simulink library "Lib_Piccolo"  (R2018b)
settings: Solver=VariableStepAuto  StartTime=0.0  StopTime=10.0  RelTol=1e-3
values from neighbouring files (symbols this model uses):
  AccelErrInt2Brakes = 0.15    [SimulationControlConfig16P.m]    (also in SimulationControlConfig16P_F0.m; SimulationControlConfig16P_F2.m; SimulationControlConfig16P_LEGACY.m; SimulationControlConfigTAILLESS.m = 0.2)
  AileronMax = 25    [SimulationControlConfig16P.m]    (also in SimulationControlConfig16P_F0.m; SimulationControlConfig16P_F2.m; SimulationControlConfig16P_LEGACY.m; SimulationControlConfigTAILLESS.m)
  AileronPower = 0.00268    [SimulationControlConfig16P.m]    (also in SimulationControlConfig16P_F0.m; SimulationControlConfig16P_F2.m; SimulationControlConfig16P_LEGACY.m; SimulationControlConfigTAILLESS.m = 0.002266)
  AileronSurfaceMax = 45    [SimulationControlConfig16P.m]    (also in SimulationControlConfig16P_F0.m; SimulationControlConfig16P_F2.m; SimulationControlConfig16P_LEGACY.m; SimulationControlConfigTAILLESS_CGAFT_F0.m = 25)
  AileronTrim = 0    [SimulationControlConfig16P.m]    (also in SimulationControlConfig16P_F0.m; SimulationControlConfig16P_F2.m; SimulationControlConfig16P_LEGACY.m; SimulationControlConfigTAILLESS.m)
  Alt = 1000 + TerrainHeight    [SimulationStateConfig.m]
  AltCruise_m = Alt * 0.3048    [SimulationControlConfig16P.m]    (also in SimulationControlConfig16P_F2.m; SimulationControlConfigTAILLESS.m = Alt/3.28084; SimulationControlConfigTAILLESS_CGAFT_F0.m = 640; SimulationControlConfigTAILLESS_CGFWD_F0.m = 640)
  AltitudeRate2PitchCmdIntegratorInit = 0.1    [SimulationControlPre.m]
  AltMax = 10000    [SimulationControlConfig16P.m]    (also in SimulationControlConfig16P_F0.m; SimulationControlConfig16P_F2.m; SimulationControlConfig16P_LEGACY.m; SimulationControlConfigTAILLESS.m)
  AltMaxAccel = 2.5    [SimulationControlConfig16P.m]    (also in SimulationControlConfig16P_F0.m = 2; SimulationControlConfig16P_F2.m = 2; SimulationControlConfig16P_LEGACY.m = 0.9; SimulationControlConfigTAILLESS.m = 2)
  AltMin = 0    [SimulationControlConfig16P.m]    (also in SimulationControlConfig16P_F0.m; SimulationControlConfig16P_F2.m; SimulationControlConfig16P_LEGACY.m; SimulationControlConfigTAILLESS.m)
  AltRateCmd2Pitch = 0.26    [SimulationControlConfig16P.m]    (also in SimulationControlConfig16P_F0.m = 0.35; SimulationControlConfig16P_F2.m = 0.35; SimulationControlConfig16P_LEGACY.m = 0.6; SimulationControlConfigTAILLESS.m = 0.9)
  AltRateError2Pitch = 0.34    [SimulationControlConfig16P.m]    (also in SimulationControlConfig16P_F0.m = 0.61; SimulationControlConfig16P_F2.m = 0.61; SimulationControlConfig16P_LEGACY.m = 0.4; SimulationControlConfigTAILLESS.m = 0.3)
  AltRateErrorInt2Pitch = 0.61    [SimulationControlConfig16P.m]    (also in SimulationControlConfig16P_F0.m = 0.28; SimulationControlConfig16P_F2.m = 0.28; SimulationControlConfig16P_LEGACY.m = 0.45; SimulationControlConfigTAILLESS.m = 0.15)
  AltRateLpfCutOff = 3    [SimulationControlConfig16P.m]    (also in SimulationControlConfig16P_F0.m; SimulationControlConfig16P_F2.m; SimulationControlConfig16P_LEGACY.m; SimulationControlConfigTAILLESS.m = 5)
  AutoNosegear2Rudder = 26    [SimulationControlConfig16P.m]    (also in SimulationControlConfig16P_F0.m; SimulationControlConfig16P_F2.m; SimulationControlConfig16P_LEGACY.m; SimulationControlConfigTAILLESS.m = 25.2)
  b = 5.54    [SimulationControlConfig16P.m]    (also in SimulationControlConfig16P_F0.m; SimulationControlConfig16P_F2.m; SimulationControlConfig16P_LEGACY.m; SimulationControlConfigTAILLESS.m = 2.37)
  Bank2AileronIntegratorInit = 0    [SimulationControlPre.m]
  BankMax_User = BankMax_User/180*pi    (= 0.610865238198)    [SimulationControlConfig16P.m]    (also in SimulationControlConfig16P_F0.m = 0.523598775598; SimulationControlConfig16P_F2.m = 0.523598775598; SimulationControlConfig16P_LEGACY.m = 0.523598775598; SimulationControlConfigTAILLESS.m = 0.558505360638)
  baseLegFlaps = 20    [SimulationControlConfig16P.m]    (also in SimulationControlConfig16P_F0.m; SimulationControlConfig16P_F2.m = 15; SimulationControlConfig16P_LEGACY.m = 0; SimulationControlConfigTAILLESS.m = 0)
  C = GeneticOpt.C    [SimulationCostFunction.m]
  c = Sw/b    (= 0.841696750903)    [SimulationControlConfig16P.m]    (also in SimulationControlConfig16P_F0.m; SimulationControlConfig16P_F2.m; SimulationControlConfig16P_LEGACY.m; SimulationControlConfigTAILLESS.m = 0.354008438819)
  cell2WheelFactorMG = 5.98    [SimulationSensorConfig16P_LEGACY.m]
  cell2WheelFactorNG = 1    [SimulationSensorConfig16P_LEGACY.m]
  cellSatMaxMG = 15000    [SimulationSensorConfig16P.m]    (also in SimulationSensorConfig16P_LEGACY.m; SimulationSensorConfigTAILLESS7P.m; SimulationSensorConfigUTAIL7P.m)
  cellSatMaxNG = 1000    [SimulationSensorConfig16P.m]    (also in SimulationSensorConfig16P_LEGACY.m; SimulationSensorConfigTAILLESS7P.m; SimulationSensorConfigUTAIL7P.m)
  cellSatMinMG = -15000    [SimulationSensorConfig16P.m]    (also in SimulationSensorConfig16P_LEGACY.m; SimulationSensorConfigTAILLESS7P.m; SimulationSensorConfigUTAIL7P.m)
  cellSatMinNG = -1000    [SimulationSensorConfig16P.m]    (also in SimulationSensorConfig16P_LEGACY.m; SimulationSensorConfigTAILLESS7P.m; SimulationSensorConfigUTAIL7P.m)
  CL_Limit = CL_Max    (= 0.54)    [SimulationControlConfig16P.m]    (also in SimulationControlConfig16P_F0.m; SimulationControlConfig16P_F2.m = 0.638; SimulationControlConfig16P_LEGACY.m; SimulationControlConfigTAILLESS.m = 0.525)
  CL_Max = 0.54    [SimulationControlConfig16P.m]    (also in SimulationControlConfig16P_F0.m; SimulationControlConfig16P_F2.m = 0.638; SimulationControlConfig16P_LEGACY.m; SimulationControlConfigTAILLESS.m = 0.525)
  CL_Max_Nom = 0.465    [SimulationControlConfig16P.m]    (also in SimulationControlConfig16P_F0.m; SimulationControlConfig16P_F2.m = 0.563; SimulationControlConfig16P_LEGACY.m; SimulationControlConfigTAILLESS.m = 0.39)
  CL_Min = 0    [SimulationControlConfig16P.m]    (also in SimulationControlConfig16P_F0.m; SimulationControlConfig16P_F2.m; SimulationControlConfig16P_LEGACY.m; SimulationControlConfigTAILLESS.m)
  ClimbMaxFraction = 0.35    [SimulationControlConfig16P.m]    (also in SimulationControlConfig16P_F0.m = 0.17; SimulationControlConfig16P_F2.m = 0.17; SimulationControlConfig16P_LEGACY.m = 0.24; SimulationControlConfigTAILLESS.m = 0.21)
  ClimboutMaxBank = 7.0    (= 7)    [SimulationControlConfig16P.m]    (also in SimulationControlConfig16P_F0.m; SimulationControlConfig16P_F2.m; SimulationControlConfig16P_LEGACY.m; SimulationControlConfigTAILLESS.m = 5)
  ClimboutTimer = 7.0    (= 7)    [SimulationControlConfig16P.m]    (also in SimulationControlConfig16P_F0.m; SimulationControlConfig16P_F2.m; SimulationControlConfig16P_LEGACY.m; SimulationControlConfigTAILLESS.m)
  dCl_per_dFlap = 0.005581818    [SimulationControlConfig16P.m]    (also in SimulationControlConfig16P_F0.m = 0; SimulationControlConfig16P_F2.m = 0.0065; SimulationControlConfig16P_LEGACY.m = 0; SimulationControlConfigTAILLESS.m = 0)
  DecelerationCmd = 3.1    [SimulationControlConfig16P.m]    (also in SimulationControlConfig16P_F0.m; SimulationControlConfig16P_F2.m; SimulationControlConfig16P_LEGACY.m; SimulationControlConfigTAILLESS.m = 0.1)
  DeRotateLogicEndTimer = abs((NoseDownLimit_Deg-1)/DeRotateRamp_Dps)    [SimulationControlConfig16P.m]    (also in SimulationControlConfig16P_F0.m; SimulationControlConfig16P_F2.m; SimulationControlConfig16P_LEGACY.m; SimulationControlConfigTAILLESS.m)
  DeRotateLogicHoldNoseUpTimer = 0.1    [SimulationControlConfig16P.m]    (also in SimulationControlConfig16P_F0.m; SimulationControlConfig16P_F2.m; SimulationControlConfig16P_LEGACY.m; SimulationControlConfigTAILLESS.m)
  DeRotateLogicTimerTimeout = 2    [SimulationControlConfig16P.m]    (also in SimulationControlConfig16P_F0.m; SimulationControlConfig16P_F2.m; SimulationControlConfig16P_LEGACY.m; SimulationControlConfigTAILLESS.m)
  DeRotateLowerCmdSaturation = 0    [SimulationControlConfig16P.m]    (also in SimulationControlConfig16P_F0.m; SimulationControlConfig16P_F2.m; SimulationControlConfig16P_LEGACY.m; SimulationControlConfigTAILLESS.m)
  DeRotateRamp_Dps = 3    [SimulationControlConfig16P.m]    (also in SimulationControlConfig16P_F0.m; SimulationControlConfig16P_F2.m; SimulationControlConfig16P_LEGACY.m; SimulationControlConfigTAILLESS.m = 8)
  DeRotateUpperCmdSaturation = 7    [SimulationControlConfig16P.m]    (also in SimulationControlConfig16P_F0.m; SimulationControlConfig16P_F2.m; SimulationControlConfig16P_LEGACY.m; SimulationControlConfigTAILLESS.m)
  DescentMaxFraction = 0.22    [SimulationControlConfig16P.m]    (also in SimulationControlConfig16P_F0.m = 0.2; SimulationControlConfig16P_F2.m = 0.2; SimulationControlConfig16P_LEGACY.m = 0.2; SimulationControlConfigTAILLESS.m = 0.17)
  DesktopSimTerrainOffset_m = 0.406    [SimulationAircraftConfig.m]
  downwindFlaps = 0    [SimulationControlConfig16P.m]    (also in SimulationControlConfig16P_F0.m; SimulationControlConfig16P_F2.m = 15; SimulationControlConfig16P_LEGACY.m; SimulationControlConfigTAILLESS.m)
  downwindSplitAil = 0    [SimulationControlConfig16P_F2.m]
  DP_init = 0.5*1.225*V_init^2    [SimulationControlConfig16P.m]    (also in SimulationControlConfig16P_F0.m; SimulationControlConfig16P_F2.m; SimulationControlConfig16P_LEGACY.m; SimulationControlConfigTAILLESS.m)
  dscNoiseMG = 1    [SimulationSensorConfig16P_LEGACY.m]
  dscNoiseNG = 0.25    [SimulationSensorConfig16P_LEGACY.m]
  DSCnumBits = 24    [SimulationSensorConfig16P.m]    (also in SimulationSensorConfig16P_LEGACY.m; SimulationSensorConfigTAILLESS7P.m; SimulationSensorConfigUTAIL7P.m)
  DSCRangeMaxMG = 15000    [SimulationSensorConfig16P.m]    (also in SimulationSensorConfig16P_LEGACY.m; SimulationSensorConfigTAILLESS7P.m; SimulationSensorConfigUTAIL7P.m)
  DSCRangeMaxNG = 1000    [SimulationSensorConfig16P.m]    (also in SimulationSensorConfig16P_LEGACY.m; SimulationSensorConfigTAILLESS7P.m; SimulationSensorConfigUTAIL7P.m)
  DSCRangeMinMG = -15000    [SimulationSensorConfig16P.m]    (also in SimulationSensorConfig16P_LEGACY.m; SimulationSensorConfigTAILLESS7P.m; SimulationSensorConfigUTAIL7P.m)
  DSCRangeMinNG = -1000    [SimulationSensorConfig16P.m]    (also in SimulationSensorConfig16P_LEGACY.m; SimulationSensorConfigTAILLESS7P.m; SimulationSensorConfigUTAIL7P.m)
  dt = DLLSim.dt    [SimulationTimeStep.m]    (also in SimulationTrim.m = 0.02)
  EarlyTouchdownThreshold = 3.0    (= 3)    [SimulationControlConfig16P.m]    (also in SimulationControlConfig16P_F0.m; SimulationControlConfig16P_F2.m; SimulationControlConfig16P_LEGACY.m; SimulationControlConfigTAILLESS.m)
  ElevatorDeflectionRate = 15    [SimulationControlConfig16P.m]    (also in SimulationControlConfig16P_F0.m; SimulationControlConfig16P_F2.m; SimulationControlConfig16P_LEGACY.m = 12; SimulationControlConfigTAILLESS.m = 5)
  ElevatorMax = 25    [SimulationControlConfig16P.m]    (also in SimulationControlConfig16P_F0.m; SimulationControlConfig16P_F2.m; SimulationControlConfig16P_LEGACY.m; SimulationControlConfigTAILLESS.m)
  ElevatorPower = -0.002209    [SimulationControlConfig16P.m]    (also in SimulationControlConfig16P_F0.m; SimulationControlConfig16P_F2.m; SimulationControlConfig16P_LEGACY.m; SimulationControlConfigTAILLESS.m = -0.002668)
  ElevatorTrim = -3.5    [SimulationControlConfig16P.m]    (also in SimulationControlConfig16P_F0.m; SimulationControlConfig16P_F2.m; SimulationControlConfig16P_LEGACY.m; SimulationControlConfigTAILLESS.m = -3)
  elevonBias = 0    [SimulationControlConfig16P.m]    (also in SimulationControlConfig16P_F0.m; SimulationControlConfig16P_F2.m; SimulationControlConfig16P_LEGACY.m; SimulationControlConfigTAILLESS.m)
  Enable_TAS_Protection = 0    [SimulationControlConfig16P.m]    (also in SimulationControlConfig16P_F0.m; SimulationControlConfig16P_F2.m; SimulationControlConfig16P_LEGACY.m; SimulationControlConfigTAILLESS.m)
  EnableCrossTrackAbort = 1    [SimulationControlConfig16P.m]    (also in SimulationControlConfigTAILLESS.m; SimulationControlConfigTAILLESS_CGAFT_F0.m; SimulationControlConfigTAILLESS_CGFWD_F0.m; SimulationControlConfigTAILLESS_CGFWD_F2.m)
  EnergyBandwidth = 0.04    [SimulationControlConfig16P.m]    (also in SimulationControlConfig16P_F0.m = 0.03; SimulationControlConfig16P_F2.m = 0.03; SimulationControlConfig16P_LEGACY.m = 0.02; SimulationControlConfigTAILLESS.m = 0.06)
  EngineLhFuelCut = 0    [SimulationAircraftConfig.m]
  EngineRhFuelCut = 0    [SimulationAircraftConfig.m]
  FastThrottleRate = 0.075    [SimulationControlConfig16P.m]    (also in SimulationControlConfig16P_F0.m = 0.05; SimulationControlConfig16P_F2.m = 0.05; SimulationControlConfig16P_LEGACY.m = 0.05; SimulationControlConfigTAILLESS.m = 0.1)
  FilterWarmUpTime = 2    [SimulationSensorConfig16P.m]    (also in SimulationSensorConfig16P_LEGACY.m; SimulationSensorConfigTAILLESS7P.m; SimulationSensorConfigUTAIL7P.m)
  finalApproachFlaps = 20    [SimulationControlConfig16P.m]    (also in SimulationControlConfig16P_F0.m; SimulationControlConfig16P_F2.m = 15; SimulationControlConfig16P_LEGACY.m = 0; SimulationControlConfigTAILLESS.m = 0)
  finalApproachSplitAil = 20    [SimulationControlConfig16P_F2.m]
  FinalDescentSlope_Deg = testPlans(testIndx).descentSlope    [SimulationControlConfig16P.m]    (also in SimulationControlConfig16P_F0.m; SimulationControlConfig16P_F2.m; SimulationControlConfig16P_LEGACY.m; SimulationControlConfigTAILLESS.m)
  flapMax = 0    [SimulationControlConfig16P.m]    (also in SimulationControlConfig16P_F0.m = 35; SimulationControlConfig16P_F2.m = 33; SimulationControlConfig16P_LEGACY.m; SimulationControlConfigTAILLESS.m)
  flapRate = 7.5    [SimulationControlConfig16P.m]    (also in SimulationControlConfig16P_F0.m; SimulationControlConfig16P_F2.m; SimulationControlConfig16P_LEGACY.m; SimulationControlConfigTAILLESS.m = 6.6)
  FlareHeight = 5    [SimulationControlConfig16P.m]    (also in SimulationControlConfig16P_F0.m; SimulationControlConfig16P_F2.m; SimulationControlConfig16P_LEGACY.m = 4.8; SimulationControlConfigTAILLESS.m = 2.75)
  FlareVerticalRate_mps = -0.4    [SimulationControlConfig16P.m]    (also in SimulationControlConfig16P_F0.m; SimulationControlConfig16P_F2.m; SimulationControlConfig16P_LEGACY.m = -0.5; SimulationControlConfigTAILLESS.m = -0.15)
  Fp_Aileron = 0.55*2*pi*RollRateLpfCutoff*dt    [SimulationControlConfig16P.m]    (also in SimulationControlConfig16P_F0.m; SimulationControlConfig16P_F2.m; SimulationControlConfig16P_LEGACY.m; SimulationControlConfigTAILLESS.m)
  Fp_Alt = 2*pi*0.55*AltBandwidth    (= 0.622035345411)    [SimulationControlConfig16P.m]    (also in SimulationControlConfig16P_F0.m; SimulationControlConfig16P_F2.m; SimulationControlConfig16P_LEGACY.m = 0.099; SimulationControlConfigTAILLESS.m = 0.207345115137)
  Fp_AltRate = 0.55*2*pi*AltRateLpfCutOff*dt    [SimulationControlConfig16P.m]    (also in SimulationControlConfig16P_F0.m; SimulationControlConfig16P_F2.m; SimulationControlConfig16P_LEGACY.m; SimulationControlConfigTAILLESS.m)
  Fp_Elevator = 0.55*2*pi*PitchRateLpfCutoff*dt    [SimulationControlConfig16P.m]    (also in SimulationControlConfig16P_F0.m; SimulationControlConfig16P_F2.m; SimulationControlConfig16P_LEGACY.m; SimulationControlConfigTAILLESS.m)
  Fp_Energy = 0.55*2*pi*EnergyBandwidth    (= 0.138230076758)    [SimulationControlConfig16P.m]    (also in SimulationControlConfig16P_F0.m = 0.103672557568; SimulationControlConfig16P_F2.m = 0.103672557568; SimulationControlConfig16P_LEGACY.m = 0.069115038379; SimulationControlConfigTAILLESS.m = 0.207345115137)
  Fp_Energy2 = 0.55*2*pi*EnergyBandwidth*dt    [SimulationControlConfig16P.m]    (also in SimulationControlConfig16P_F0.m; SimulationControlConfig16P_F2.m; SimulationControlConfig16P_LEGACY.m; SimulationControlConfigTAILLESS.m)
  Fp_Pitch = 0.55*2*pi*PitchBandwidth    (= 2.45358386245)    [SimulationControlConfig16P.m]    (also in SimulationControlConfig16P_F0.m; SimulationControlConfig16P_F2.m = 1.72787595947; SimulationControlConfig16P_LEGACY.m = 3.11017672705; SimulationControlConfigTAILLESS.m = 1.55508836353)
  Fp_Pitch_2 = 0.55*2*pi*PitchBandwidth*dt    [SimulationControlConfig16P.m]    (also in SimulationControlConfig16P_F0.m; SimulationControlConfig16P_F2.m; SimulationControlConfig16P_LEGACY.m; SimulationControlConfigTAILLESS.m)
  Fp_Roll = RollBandwidth^2    (= 1.69)    [SimulationControlConfig16P.m]    (also in SimulationControlConfig16P_F0.m = 1.44; SimulationControlConfig16P_F2.m = 1.44; SimulationControlConfig16P_LEGACY.m = 1.44; SimulationControlConfigTAILLESS.m = 1.21)
  Fp_Rudder = 0.55*2*pi*YawRateLpfCutoff*dt    [SimulationControlConfig16P.m]    (also in SimulationControlConfig16P_F0.m; SimulationControlConfig16P_F2.m; SimulationControlConfig16P_LEGACY.m; SimulationControlConfigTAILLESS.m)
  Fp_TAS = 0.55*2*pi*TASBandwidth    (= 0.103672557568)    [SimulationControlConfig16P.m]    (also in SimulationControlConfig16P_F0.m; SimulationControlConfig16P_F2.m; SimulationControlConfig16P_LEGACY.m; SimulationControlConfigTAILLESS.m = 0.172787595947)
  Fp_TAS_Filter = 2*pi*TasLpfCutoff*dt    [SimulationControlConfig16P.m]    (also in SimulationControlConfig16P_F0.m; SimulationControlConfig16P_F2.m; SimulationControlConfig16P_LEGACY.m; SimulationControlConfigTAILLESS.m)
  Fp_Turn = 0.55*2*pi*TurnErrLPFcutoff    (= 0.172787595947)    [SimulationControlConfig16P.m]    (also in SimulationControlConfig16P_F0.m = 0.0345575191895; SimulationControlConfig16P_F2.m = 0.0345575191895; SimulationControlConfig16P_LEGACY.m = 0.0345575191895; SimulationControlConfigTAILLESS.m)
  Fp_TurnDerr = 0.55*2*pi*TurnDerivativeLPFcutoff    (= 0.172787595947)    [SimulationControlConfig16P.m]    (also in SimulationControlConfig16P_F0.m = 0.0345575191895; SimulationControlConfig16P_F2.m = 0.0345575191895; SimulationControlConfig16P_LEGACY.m = 0.0345575191895; SimulationControlConfigTAILLESS.m)
  FTV = 3    [SimulationAircraftConfig.m]
  ftvStaticPositionError = 1/1.18    (= 0.847457627119)    [SimulationSensorConfig16P.m]    (also in SimulationSensorConfig16P_LEGACY.m; SimulationSensorConfigTAILLESS7P.m = 1; SimulationSensorConfigUTAIL7P.m = 1)
  g = 9.81    [SimulationStateConfig.m]
  goAroundSplitAil = 0    [SimulationControlConfig16P_F2.m]
  GustSpd_Kts = testPlans(testIndx).gustSpd    [SimulationStateConfig.m]
  GustTriggerVal = testPlans(testIndx).gustTriggerVal    [SimulationStateConfig.m]
  HeadingErr2TurnRate = 0.5    [SimulationControlConfig16P.m]    (also in SimulationControlConfig16P_F0.m; SimulationControlConfig16P_F2.m; SimulationControlConfig16P_LEGACY.m; SimulationControlConfigTAILLESS.m)
  HeadingErrDer2TurnRate = 0.3    [SimulationControlConfig16P.m]    (also in SimulationControlConfig16P_F0.m; SimulationControlConfig16P_F2.m; SimulationControlConfig16P_LEGACY.m; SimulationControlConfigTAILLESS.m)
  IASbounce = IASstall*0.8    [SimulationControlPre.m]
  IAScruiseCMD = sqrt(2*m*9.81/(1.225*Sw*CL_cruise))    [SimulationControlConfig16P.m]    (also in SimulationControlConfig16P_F0.m; SimulationControlConfig16P_F2.m; SimulationControlConfig16P_LEGACY.m; SimulationControlConfigTAILLESS.m)
  IASfinalCMD = 1.12 * IASmin    [SimulationControlConfig16P.m]    (also in SimulationControlConfig16P_F0.m = 1.14 * IASmin; SimulationControlConfig16P_F2.m = 1.10 * IASmin; SimulationControlConfig16P_LEGACY.m = 1.10 * IASmin; SimulationControlConfigTAILLESS.m = 1.14 * IASmin)
  IASflareCMD = IASstall    [SimulationControlConfig16P.m]    (also in SimulationControlConfig16P_F0.m; SimulationControlConfig16P_F2.m; SimulationControlConfig16P_LEGACY.m; SimulationControlConfigTAILLESS.m)
  IASmax = 64    [SimulationControlConfig16P.m]    (also in SimulationControlConfig16P_F0.m = 46; SimulationControlConfig16P_F2.m = 52; SimulationControlConfig16P_LEGACY.m = 46; SimulationControlConfigTAILLESS.m = 38.9)
  IASmin = sqrt(2*m*9.81/(1.225*Sw*0.9*CL_Max_Nom))    [SimulationControlConfig16P.m]    (also in SimulationControlConfig16P_F0.m; SimulationControlConfig16P_F2.m; SimulationControlConfig16P_LEGACY.m; SimulationControlConfigTAILLESS.m)
  IASshortCMD = IASstall    [SimulationControlConfig16P.m]    (also in SimulationControlConfig16P_F0.m; SimulationControlConfig16P_F2.m; SimulationControlConfig16P_LEGACY.m; SimulationControlConfigTAILLESS.m)
  IASstall = sqrt(2*m*9.81/(1.225*Sw*CL_Max))    [SimulationControlConfig16P.m]    (also in SimulationControlConfig16P_F0.m; SimulationControlConfig16P_F2.m; SimulationControlConfig16P_LEGACY.m; SimulationControlConfigTAILLESS.m)
  inFlight = 1    [SimulationControlConfig16P.m]    (also in SimulationControlConfigTAILLESS.m; SimulationControlConfigTAILLESS_CGAFT_F0.m; SimulationControlConfigTAILLESS_CGFWD_F0.m; SimulationControlConfigTAILLESS_CGFWD_F2.m)
  JetCatOffset = 5    [SimulationControlConfig16P.m]    (also in SimulationControlConfig16P_F0.m; SimulationControlConfig16P_F2.m; SimulationControlConfig16P_LEGACY.m)
  LaunchRollingElevator = -1.5    [SimulationControlConfig16P.m]    (also in SimulationControlConfig16P_F0.m; SimulationControlConfig16P_F2.m = 1.25; SimulationControlConfig16P_LEGACY.m; SimulationControlConfigTAILLESS.m = 1)
  ldg_NosegearMax = 10    [SimulationControlConfig16P.m]    (also in SimulationControlConfig16P_F0.m; SimulationControlConfig16P_F2.m; SimulationControlConfig16P_LEGACY.m; SimulationControlConfigTAILLESS.m)
  ldg_TrackVyErrInt2Nosegear = 0.1250    (= 0.125)    [SimulationControlConfig16P.m]    (also in SimulationControlConfig16P_F0.m; SimulationControlConfig16P_F2.m; SimulationControlConfig16P_LEGACY.m; SimulationControlConfigTAILLESS.m = 0.00714285714286)
  ldg_TrackVyErrPro2Nosegear = 0.35    [SimulationControlConfig16P.m]    (also in SimulationControlConfig16P_F0.m; SimulationControlConfig16P_F2.m; SimulationControlConfig16P_LEGACY.m; SimulationControlConfigTAILLESS.m = 0.0546666666667)
  ldg_TrackY2Vy = 0.07    [SimulationControlConfig16P.m]    (also in SimulationControlConfig16P_F0.m; SimulationControlConfig16P_F2.m; SimulationControlConfig16P_LEGACY.m; SimulationControlConfigTAILLESS.m = 0.17)
  ldg_Vy2NosegearScalingPower = 1.075    [SimulationControlConfig16P.m]    (also in SimulationControlConfig16P_F0.m; SimulationControlConfig16P_F2.m; SimulationControlConfig16P_LEGACY.m; SimulationControlConfigTAILLESS.m = 0.6)
  ldg_Y2VyScalingPower = 0.175    [SimulationControlConfig16P.m]    (also in SimulationControlConfig16P_F0.m; SimulationControlConfig16P_F2.m; SimulationControlConfig16P_LEGACY.m; SimulationControlConfigTAILLESS.m = 0)
  ldg_YawRate2Nosegear = 0.175    [SimulationControlConfig16P.m]    (also in SimulationControlConfig16P_F0.m; SimulationControlConfig16P_F2.m; SimulationControlConfig16P_LEGACY.m; SimulationControlConfigTAILLESS.m = 0.065)
  LiftSlope = 0.064285    [SimulationControlConfig16P.m]    (also in SimulationControlConfig16P_F0.m; SimulationControlConfig16P_F2.m; SimulationControlConfig16P_LEGACY.m; SimulationControlConfigTAILLESS.m = 0.058631)
  LPFaileronInit = 0    [SimulationControlPre.m]
  LPFclestInit = 0    [SimulationControlPre.m]
  LPFenergyFFInit = 0    [SimulationControlPre.m]
  ... (+122 more)
undefined symbols (not defined in the file or in its folder): abortFlag, alphaHPF, apmDelay, BRWNOUT, CRAWOR, CRAWUR, DiscIntNeverNeededParam, DLLSim, DLLSimStep, ECOMOR, ECOMUR, Fp_Tas, GustTrigger_HeightAgl_m, IPSTAT, LCINTEG, Ldg_Persist_Time, LOWER_FLAGS, MSG_ENABLE, NoiseStd, OLDVAL, OVERRIDE_ENABLE, OVERRIDE_VALUE, REBOOT, reversionEnable, revIASMax, revIASMin, revPitchMax, revPitchMin, revPitchRateMax, revRollMax, revRollRateMax, SAMPLE, SCALON, SensorModel, sigbuilder_block, Sim_Vx, Sim_Vy, Sim_Vz, Sim_Xpos, Sim_Ypos, Sim_Zpos, SYSOR, SYSUR, TARE, TEMPOR, TEMPUR, testIndx, testPlan, testPlans, Trim_piccoloInCmd, Trim_REFSI_FD_IN_nmodeCgShifterCmd_Flag, Trim_REFSI_FD_IN_nmodeCgShifterCmd_Ft, Trim_REFSI_FD_IN_nmodeCgShifterCmdType, Trim_REFSI_FD_IN_nmodeCgShifterNRCActive, Trim_REFSI_FD_IN_nmodeFlapLhIBCmd_Deg, Trim_REFSI_FD_IN_nmodeFlapLhOBCmd_Deg, Trim_REFSI_FD_IN_nmodeFlapRhIBCmd_Deg, Trim_REFSI_FD_IN_nmodeFlapRhOBCmd_Deg, Trim_REFSI_FD_IN_nmodeSlatLhCmd_Deg ... (+11)
libraries: simulink x1237, $bdroot x179, aerolibconvert2 x63, dspswit3 x25, aerolibatmos2 x5, simulink_extras x4, dsparch4 x2, Lib_Piccolo_Alt x2, eeGeneralControl x1, dspindex x1
(part 5 of 74)

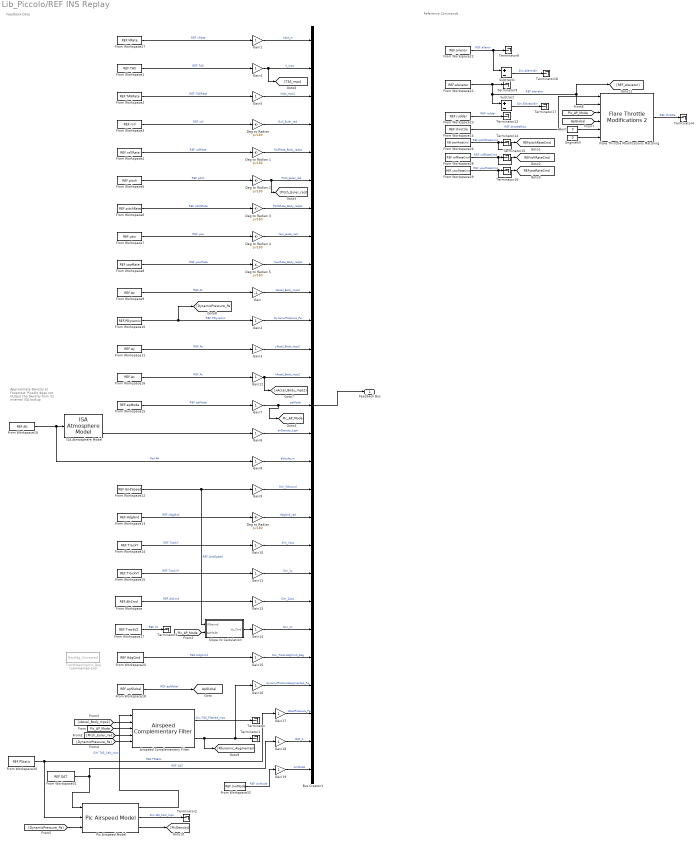
== system Lib_Piccolo/REF INS Replay ==
  note: Feedback Data
  note: Approximate Density at Foremost. Piccolo does not Output the Density from its internal ISA lookup
  note: Reference Commands
  Abort : Constant  Value=0
  Airspeed Complementary Filter : $bdroot/Airspeed Complementary Filter  SystemSampleTime=-1
  Bus Creator1 : BusCreator  Inputs=27
  Deg to Radian : Gain  Gain=pi/180
  Deg to Radian {,1..5} (6 alike) : Gain  Gain=pi/180
  EngineKill : Constant  Value=0
  Flare Throttle Modifications Matching : $bdroot/Throttle Control (Alt Mode)/Flare Throttle Modifications 2  SystemSampleTime=-1
  From Workspace : FromWorkspace  VariableName=REF.AltCmd  SampleTime=0
  From Workspace1 : FromWorkspace  VariableName=REF.TAS  SampleTime=0
  From Workspace10 : FromWorkspace  VariableName=REF.PDynamic  SampleTime=0
  From Workspace11 : FromWorkspace  VariableName=REF.Ay  SampleTime=0
  From Workspace12 : FromWorkspace  VariableName=REF.GndSpeed  SampleTime=0
  From Workspace13 : FromWorkspace  VariableName=REF.HdgGnd  SampleTime=0
  From Workspace14 : FromWorkspace  VariableName=REF.TrackY  SampleTime=0
  From Workspace15 : FromWorkspace  VariableName=REF.TrackVY  SampleTime=0
  From Workspace16 : FromWorkspace  VariableName=REF.Ax  SampleTime=0
  From Workspace17 : FromWorkspace  VariableName=REF.TrackVZ  SampleTime=0
  From Workspace18 : FromWorkspace  VariableName=REF.apGlobal  SampleTime=0
  From Workspace19 : FromWorkspace  VariableName=REF.Alt  SampleTime=0
  From Workspace2 : FromWorkspace  VariableName=REF.TASRate  SampleTime=0
  From Workspace20 : FromWorkspace  VariableName=REF.HdgCmd  SampleTime=0
  From Workspace21 : FromWorkspace  VariableName=REF.elevator  SampleTime=0
  From Workspace22 : FromWorkspace  VariableName=REF.aileron  SampleTime=0
  From Workspace23 : FromWorkspace  VariableName=REF.rudder  SampleTime=0
  From Workspace24 : FromWorkspace  VariableName=REF.throttle  SampleTime=0
  From Workspace25 : FromWorkspace  VariableName=REF.apMode  SampleTime=0
  From Workspace26 : FromWorkspace  VariableName=REF.pitchRateCmd  SampleTime=0
  From Workspace27 : FromWorkspace  VariableName=REF.VRate  SampleTime=0
  From Workspace28 : FromWorkspace  VariableName=REF.rollRateCmd  SampleTime=0
  From Workspace29 : FromWorkspace  VariableName=REF.yawRateCmd  SampleTime=0
  From Workspace3 : FromWorkspace  VariableName=REF.roll  SampleTime=0
  From Workspace30 : FromWorkspace  VariableName=REF.PStatic  SampleTime=0
  From Workspace31 : FromWorkspace  VariableName=REF.OAT  SampleTime=0
  From Workspace32 : FromWorkspace  VariableName=REF.lonMode  SampleTime=0
  From Workspace4 : FromWorkspace  VariableName=REF.rollRate  SampleTime=0
  From Workspace5 : FromWorkspace  VariableName=REF.pitch  SampleTime=0
  From Workspace6 : FromWorkspace  VariableName=REF.pitchRate  SampleTime=0
  From Workspace7 : FromWorkspace  VariableName=REF.yaw  SampleTime=0
  From Workspace8 : FromWorkspace  VariableName=REF.yawRate  SampleTime=0
  From Workspace9 : FromWorkspace  VariableName=REF.Az  SampleTime=0
  Gain : Gain  Gain=-1
  Gain{1..19} (19 alike) : Gain
  ISA Atmosphere Model : aerolibatmos2/ISA Atmosphere Model  custom=off  g=9.80665  gamma=1.4  R=287.0531  L=0.0065  h_trop=11000  h_strat=20000  rho0=1.225  P0=101325  T0=288.15  h0=0
      settings: SourceProductName=Aerospace Blockset
  Pic Airspeed Model : $bdroot/Pic Airspeed Model  correction=1
  Slope Vz Calculation : Subsystem
  Subtract : Sum  Inputs=+-
  Subtract1 : Sum  Inputs=+-
  Terminator{,1..4,8..9,12,14..18} (13 alike) : Terminator
  TrackHeadingInit_Deg : Constant  Commented=on  Value=RwyHdg_Corrected
  Feedback Bus : Outport
  tag scope: ApGlobal=global, Pic_AP_Mode=global, REFpitchRateCmd=global, REFrollRateCmd=global, REFyawRateCmd=global
  wires:
  Deg to Radian 2/1 -> [Pitch_Euler_rad], Bus Creator1/6  "Pitch_Euler_rad"
  Deg to Radian 3/1 -> Bus Creator1/7  "PitchRate_Body_radps"
  Gain/1 -> Bus Creator1/10  "zAccel_Body_mps2"
  Deg to Radian 5/1 -> Bus Creator1/9  "YawRate_Body_radps"
  Deg to Radian 4/1 -> Bus Creator1/8  "Yaw_Euler_rad"
  Bus Creator1/1 -> Feedback Bus/1
  Gain3/1 -> Bus Creator1/12  "yAccel_Body_mps2"
  Gain1/1 -> Bus Creator1/1  "hdot_m"
  Gain4/1 -> [TAS_mps], Bus Creator1/2  "V_mps"
  Gain5/1 -> Bus Creator1/3  "Vdot_mps2"
  "Deg to Radian "/1 -> Bus Creator1/4  "Roll_Euler_rad"
  Deg to Radian 1/1 -> Bus Creator1/5  "RollRate_Body_radps"
  Gain6/1 -> Bus Creator1/15  "airDensity_kgm"
  From Workspace27/1 -> Gain1/1  "REF.vRate"
  From Workspace2/1 -> Gain5/1  "REF.TASRate"
  From Workspace3/1 -> "Deg to Radian "/1  "REF.roll"
  From Workspace4/1 -> Deg to Radian 1/1  "REF.rollRate"
  From Workspace5/1 -> Deg to Radian 2/1  "REF.pitch"
  From Workspace6/1 -> Deg to Radian 3/1  "REF.pitchRate"
  From Workspace7/1 -> Deg to Radian 4/1  "REF.yaw"
  From Workspace8/1 -> Deg to Radian 5/1  "REF.yawRate"
  From Workspace9/1 -> Gain/1  "REF.Az"
  From Workspace10/1 -> [DynamicPressure_Pa], Gain2/1  "REF.PDynamic"
  From Workspace11/1 -> Gain3/1  "REF.Ay"
  ISA Atmosphere Model/4 -> Gain6/1
  From Workspace19/1 -> Gain8/1, ISA Atmosphere Model/1  "Ref.Alt"
  Gain7/1 -> [Pic_AP_Mode], Bus Creator1/14  "apMode"
  From Workspace25/1 -> Gain7/1  "REF.apMode"
  Gain8/1 -> Bus Creator1/16  "altitude_m"
  Gain9/1 -> Bus Creator1/17  "Sim_VGround"
  From Workspace12/1 -> Slope Vz Calculation/1(VGround), Gain9/1  "REF.GndSpeed"
  From Workspace13/1 -> Deg to Radian/1  "REF.HdgGnd"
  Deg to Radian/1 -> Bus Creator1/18  "HdgGnd_rad"
  From Workspace1/1 -> Gain4/1  "REF.TAS"
  From Workspace14/1 -> Gain10/1  "REF.TrackY"
  Gain10/1 -> Bus Creator1/19  "Sim_Ypos"
  From Workspace15/1 -> Gain11/1  "REF.TrackVY"
  Gain11/1 -> Bus Creator1/20  "Sim_Vy"
  From Workspace16/1 -> Gain12/1  "REF.Ax"
  Gain12/1 -> [xAccel_Body_mps2], Bus Creator1/13  "xAccel_Body_mps2"
  From Workspace/1 -> Gain13/1  "REF.AltCmd"
  Gain13/1 -> Bus Creator1/21  "Sim_Zpos"
  Gain14/1 -> Bus Creator1/22  "Sim_Vz"
  From Workspace17/1 -> Terminator3/1  "REF.Vz"
  From Workspace18/1 -> [ApGlobal]  "REF.apGlobal"
  Gain15/1 -> Bus Creator1/23  "Sim_TrackHdgCmd_Deg"
  From Workspace20/1 -> Gain15/1  "REF.HdgCmd"
  [Pic_AP_Mode] -> Airspeed Complementary Filter/3
  [Pitch_Euler_rad] -> Airspeed Complementary Filter/4
  [xAccel_Body_mps2] -> Airspeed Complementary Filter/2
  Airspeed Complementary Filter/1 -> Terminator/1  "Sim.TAS_Filtered_mps"
  [DynamicPressure_Pa] -> Airspeed Complementary Filter/5
  Airspeed Complementary Filter/2 -> [Pdynamic_Augmented], Gain16/1, Terminator1/1
  Gain16/1 -> Bus Creator1/24  "dynamicPressureAugmented_Pa"
  Pic Airspeed Model/1 -> Airspeed Complementary Filter/1  "Sim.TAS_Calc_mps"
  Pic Airspeed Model/2 -> Terminator2/1  "Sim.IAS_Calc_mps"
  [DynamicPressure_Pa] -> Pic Airspeed Model/3
  From Workspace30/1 -> Pic Airspeed Model/2, Gain17/1  "REF.PStatic"
  Gain17/1 -> Bus Creator1/25  "staticPressure_Pa"
  From Workspace31/1 -> Pic Airspeed Model/1, Gain18/1  "REF.OAT"
  Gain18/1 -> Bus Creator1/26  "OAT_C"
  Gain2/1 -> Bus Creator1/11  "DynamicPressure_Pa"
  Pic Airspeed Model/3 -> [PicDensity]
  Slope Vz Calculation/1(Vz_Cmd) -> Gain14/1
  [Pic_AP_Mode] -> Slope Vz Calculation/2(apMode)
  From Workspace24/1 -> Flare Throttle Modifications Matching/1  "REF.throttleRaw"
  Abort/1 -> Flare Throttle Modifications Matching/5
  From Workspace26/1 -> [REFpitchRateCmd], Terminator14/1  "REF.pitchRateCmd"
  From Workspace23/1 -> Terminator12/1  "REF.rudder"
  From Workspace29/1 -> [REFyawRateCmd], Terminator16/1  "REF.yawRateCmd"
  Subtract/1 -> Terminator17/1  "Sim.ElevatorErr"
  [Pic_AP_Mode] -> Flare Throttle Modifications Matching/3
  EngineKill/1 -> Flare Throttle Modifications Matching/6
  From Workspace22/1 -> Terminator8/1, Subtract1/1  "REF.aileron"
  Subtract1/1 -> Terminator18/1  "Sim.AileronErr"
  From Workspace21/1 -> Terminator9/1, [REF_elevator], Flare Throttle Modifications Matching/2, Subtract/1  "REF.elevator"
  Flare Throttle Modifications Matching/1 -> Terminator4/1  "REF.throttle"
  From Workspace28/1 -> [REFrollRateCmd], Terminator15/1  "REF.rollRateCmd"
  [ApGlobal] -> Flare Throttle Modifications Matching/4
  From Workspace32/1 -> Gain19/1  "REF.lonMode"
  Gain19/1 -> Bus Creator1/27  "lonMode"

== system Lib_Piccolo/Sliding Window Maximum ==
  note: Insert new element
  note: Remove last element
  note: Define dimensions
      | (initial conditions)
  windowInput : Inport
  IC : InitialCondition  Value=[zeros(N,1)]
  Max : MinMax  Function=max
  Memory : Memory
  Mux : Mux  Inputs=2
  Variable Selector : dspindex/Variable Selector  NumInputs=1  rowsOrCols=Rows  IdxMode=Fixed  Elements=1:N-1  ZerOneIdxMode=One-based  errmode=Clip Index  FillMode=on  FillValues=0
  windowMax : Outport
  wires:
  Memory/1 -> IC/1
  Mux/1 -> Max/1, Memory/1
  windowInput/1 -> Mux/1
  Variable Selector/1 -> Mux/2
  IC/1 -> Variable Selector/1
  Max/1 -> windowMax/1

== system Lib_Piccolo/Steering Controller Landing ==
  Y command : Inport
  Feedback : Inport  Port=2
  Bus Selector : BusSelector  OutputSignals=Sim_VGround,Sim_Ypos,Sim_Vy,YawRate_Body_radps
  Constant : Constant  Value=0
  Constant1 : Constant  Value=0
  Gain3 : Gain  Gain=1/4
  Gain4 : Gain  Gain=-1
  Integrator1 : Integrator  ExternalReset=level
  NOT : Logic  Operator=NOT  IconShape=distinctive  AllPortsSameDT=off  OutDataTypeStr=boolean
  "Nosegear rudder mixer " : Subsystem
  Nosegear scaling based on ground speed : Subsystem
  Product2 : Product
  Product3 : Product
  Saturation Dynamic1 : simulink/Discontinuities/Saturation Dynamic  OutMin=[]  OutMax=[]  OutDataTypeStr=Inherit: Same as second input  OutDataType=fixdt(1, 16)  OutScaling=2^-10  DoSatur=off
  Sum4 : Sum  Inputs=|++
  Sum5 : Sum  Inputs=|+-
  Sum6 : Sum  Inputs=+-|
  Sum7 : Sum  Inputs=|+-
  Switch : Switch  Criteria=u2 > Threshold  Threshold=1.5
  Switch1 : Switch  Criteria=u2 > Threshold  Threshold=1.5
  "Track Vy error integral to nosegear " : Gain  Gain=ldg_TrackVyErrInt2Nosegear
  "Track Vy error to nosegear " : Gain  Gain=ldg_TrackVyErrPro2Nosegear
  Track Y to Vy : Gain  Gain=ldg_TrackY2Vy
  Vy scaling based on ground speed : Subsystem
  Vy to nosegear scaling power : Constant  Value=ldg_Vy2NosegearScalingPower
  "Y to Vy scaling power " : Constant  Value=ldg_Y2VyScalingPower
  Yaw rate to nosegear : Gain  Gain=ldg_YawRate2Nosegear
  Rudder_Deg : Outport
  Nosegear_Deg : Outport  Port=2
  wires:
  Y command/1 -> Sum6/1  "Sim.YCmd"
  Feedback/1 -> Bus Selector/1
  "Nosegear rudder mixer "/1(Nosegear command) -> Nosegear_Deg/1  "Sim.NosegearCmd"
  "Y to Vy scaling power "/1 -> Vy scaling based on ground speed/2(Y to Vy scaling power)
  Product2/1 -> Saturation Dynamic1/2
  Gain3/1 -> Saturation Dynamic1/1, Gain4/1
  Constant/1 -> Switch/3
  "Track Vy error integral to nosegear "/1 -> Sum4/2  "Ki_Vy"
  Yaw rate to nosegear/1 -> Sum5/2  "Sim.YawRate2Nosegear"
  "Track Vy error to nosegear "/1 -> Sum4/1  "Kp_Vy"
  Switch1/1 -> Gain3/1
  Switch/1 -> "Nosegear rudder mixer "/1("Desired nosegear ")
  Sum5/1 -> Switch/1
  Saturation Dynamic1/1 -> Sum7/1  "Sim.VyCmd"
  Nosegear scaling based on ground speed/1(nosegear scalar) -> Product3/1  "Sim.NosegearScalar"
  Bus Selector/1 -> Nosegear scaling based on ground speed/1(Ground Speed), Switch/2, Vy scaling based on ground speed/1(Ground Speed), Switch1/2, Switch1/1  "<Sim_VGround>"
  Vy scaling based on ground speed/1(Vy Scalar) -> Product2/1  "Sim.Vy Scalar"
  Constant1/1 -> Switch1/3
  Vy to nosegear scaling power/1 -> Nosegear scaling based on ground speed/2("Vy to nosegear scaling ")
  Gain4/1 -> Saturation Dynamic1/3
  Integrator1/1 -> "Track Vy error integral to nosegear "/1
  Track Y to Vy/1 -> Product2/2
  Sum4/1 -> Product3/2
  Bus Selector/3 -> Sum7/2  "<Sim_Vy>"
  Bus Selector/2 -> Sum6/2  "<Sim_Ypos>"
  Product3/1 -> Sum5/1
  "Nosegear rudder mixer "/2(Rudder command) -> Rudder_Deg/1  "Sim.RudderCmd"
  Sum6/1 -> Track Y to Vy/1  "TrackY Error"
  Sum7/1 -> "Track Vy error to nosegear "/1, Integrator1/1  "Sim.Vy Error"
  Bus Selector/4 -> Yaw rate to nosegear/1  "<YawRate_Body_radps>"
  [Rollout_Flag] -> NOT/1
  NOT/1 -> Integrator1/2

== system Lib_Piccolo/Steering Controller Selection ==
  Rollout Rudder In : Inport
  Rollout NG In : Inport  Port=2
  Transition Rudder In : Inport  Port=3
  Transition NG In : Inport  Port=4
  Switch : Switch  Threshold=5
  Switch1 : Switch  Threshold=5
  Rudder_Deg : Outport
  Nosegear_Deg : Outport  Port=2
  wires:
  [Pic_AP_Mode] -> Switch1/2, Switch/2
  Rollout Rudder In/1 -> Switch/1  "Rollout_Rud"
  Transition Rudder In/1 -> Switch/3  "Transition_Rud"
  Switch/1 -> Rudder_Deg/1
  Switch1/1 -> Nosegear_Deg/1
  Rollout NG In/1 -> Switch1/1  "Rollout_NG"
  Transition NG In/1 -> Switch1/3  "Transition_NG"

== system Lib_Piccolo/Steering Controller Transition ==
  Y command : Inport
  Feedback : Inport  Port=2
  AND : Logic  IconShape=distinctive  AllPortsSameDT=off  OutDataTypeStr=boolean
  Abs : Abs
  Bus Selector : BusSelector  OutputSignals=Sim_VGround,Sim_Ypos,Sim_Vy,YawRate_Body_radps
  Compare To Constant : simulink/Logic and Bit Operations/Compare To Constant  relop=>=  const=MaxCrossError  OutDataTypeStr=boolean
  Compare To Constant1 : simulink/Logic and Bit Operations/Compare To Constant  relop===  const=1  OutDataTypeStr=boolean
  Constant : Constant  Value=0
  Constant1 : Constant  Value=0
  Gain3 : Gain  Gain=1/4
  Gain4 : Gain  Gain=-1
  Integrator1 : Integrator  ExternalReset=level
  "Nosegear rudder mixer " : Subsystem
  Nosegear scaling based on ground speed : Subsystem
  Product2 : Product
  Product3 : Product
  Saturation Dynamic1 : simulink/Discontinuities/Saturation Dynamic  OutMin=[]  OutMax=[]  OutDataTypeStr=Inherit: Same as second input  OutDataType=fixdt(1, 16)  OutScaling=2^-10  DoSatur=off
  Sum4 : Sum  Inputs=|++
  Sum5 : Sum  Inputs=|+-
  Sum6 : Sum  Inputs=+-|
  Sum7 : Sum  Inputs=|+-
  Switch : Switch  Criteria=u2 > Threshold  Threshold=1.5
  Switch1 : Switch  Criteria=u2 > Threshold  Threshold=1.5
  "Track Vy error integral to nosegear " : Gain  Gain=TrackVyErrInt2Nosegear
  "Track Vy error to nosegear " : Gain  Gain=TrackVyErrPro2Nosegear
  Track Y to Vy : Gain  Gain=TrackY2Vy
  Vy scaling based on ground speed : Subsystem
  Vy to nosegear scaling power : Constant  Value=Vy2NosegearScalingPower
  "Y to Vy scaling power " : Constant  Value=Y2VyScalingPower
  Yaw rate to nosegear : Gain  Gain=YawRate2Nosegear
  Rudder_Deg : Outport
  Nosegear_Deg : Outport  Port=2
  tag scope: Flag_CrossTrackAbort=global
  wires:
  Y command/1 -> Sum6/1  "Sim.YCmd"
  Feedback/1 -> Bus Selector/1
  "Nosegear rudder mixer "/1(Nosegear command) -> Nosegear_Deg/1  "Sim.NosegearCmd"
  "Y to Vy scaling power "/1 -> Vy scaling based on ground speed/2(Y to Vy scaling power)
  Product2/1 -> Saturation Dynamic1/2
  Gain3/1 -> Saturation Dynamic1/1, Gain4/1
  Constant/1 -> Switch/3
  "Track Vy error integral to nosegear "/1 -> Sum4/2  "Ki_Vy"
  Yaw rate to nosegear/1 -> Sum5/2  "Sim.YawRate2Nosegear"
  "Track Vy error to nosegear "/1 -> Sum4/1  "Kp_Vy"
  Switch1/1 -> Gain3/1
  Switch/1 -> "Nosegear rudder mixer "/1("Desired nosegear ")
  Sum5/1 -> Switch/1
  Saturation Dynamic1/1 -> Sum7/1  "Sim.VyCmd"
  Nosegear scaling based on ground speed/1(nosegear scalar) -> Product3/1  "Sim.NosegearScalar"
  Bus Selector/1 -> Switch/2, Nosegear scaling based on ground speed/1(Ground Speed), Vy scaling based on ground speed/1(Ground Speed), Switch1/2, Switch1/1  "<Sim_VGround>"
  Vy scaling based on ground speed/1(Vy Scalar) -> Product2/1  "Sim.Vy Scalar"
  Constant1/1 -> Switch1/3
  Vy to nosegear scaling power/1 -> Nosegear scaling based on ground speed/2("Vy to nosegear scaling ")
  Gain4/1 -> Saturation Dynamic1/3
  Integrator1/1 -> "Track Vy error integral to nosegear "/1
  Track Y to Vy/1 -> Product2/2
  Sum4/1 -> Product3/2
  Bus Selector/3 -> Sum7/2  "<Sim_Vy>"
  Bus Selector/2 -> Sum6/2  "<Sim_Ypos>"
  Product3/1 -> Sum5/1
  "Nosegear rudder mixer "/2(Rudder command) -> Rudder_Deg/1  "Sim.RudderCmd"
  Sum6/1 -> Abs/1, Track Y to Vy/1  "TrackY Error"
  Sum7/1 -> "Track Vy error to nosegear "/1, Integrator1/1  "Sim.Vy Error"
  Bus Selector/4 -> Yaw rate to nosegear/1  "<YawRate_Body_radps>"
  [Rollout_Flag] -> Integrator1/2
  Abs/1 -> Compare To Constant/1
  Compare To Constant/1 -> AND/2
  [Pic_AP_Mode] -> Compare To Constant1/1
  AND/1 -> [Flag_CrossTrackAbort]  "Flag_CrossTrackAbort"
  Compare To Constant1/1 -> AND/1

== system Lib_Piccolo/TLA Selection ==
  Airspeed_TLA : Inport
  Alt_TLA : Inport  Port=2
  Rate Limiter : RateLimiter  RisingSlewLimit=ThrottleRateMax  FallingSlewLimit=-ThrottleRateMax  SampleTimeMode=inherited
  Switch4 : Switch  Criteria=u2 > Threshold
  Sim_ThrottleCmd : Outport
  wires:
  [Flag_TAS_Priority] -> Switch4/2
  Alt_TLA/1 -> Switch4/3
  Airspeed_TLA/1 -> Switch4/1
  Switch4/1 -> Rate Limiter/1
  Rate Limiter/1 -> Sim_ThrottleCmd/1

== system Lib_Piccolo/Throttle Control (Airspeed Mode) ==
  hCmd : Inport
  Vcmd : Inport  Port=2
  Feedback Bus : Inport  Port=3
  " " : Constant  Value=ThrottleTrim
  " TLASaturation 1" : Saturate  UpperLimit=ThrottleMax  LowerLimit=ThrottleMin  LinearizeAsGain=off
  "1/ MaxEnginePower " : Gain  Gain=1/MaxEnginePower
  1st Order Reference Model : Subsystem
  AND : Logic  IconShape=distinctive  AllPortsSameDT=off  OutDataTypeStr=boolean
  AND1 : Logic  IconShape=distinctive  AllPortsSameDT=off  OutDataTypeStr=boolean
  Bus Selector1 : BusSelector  OutputSignals=V_mps,hdot_m,Vdot_mps2,altitude_m
  Constant : Constant  Value=ThrottleMax
  Constant1 : Constant  Value=ThrottleMin
  Constant3 : Constant  Value=ThrottleRateMax
  Constant5 : Constant  Value=100
  Divide : Product  Inputs=**
  Gain : Gain  Gain=m/2
  Gain1 : Gain  Gain=m
  Gain2 : Gain  Gain=m*g
  Gain3 : Gain  Gain=m/2
  Gain4 : Gain  Gain=-1
  Gain6 : Gain  Gain=m*g
  Gain7 : Gain  Gain=m*g
  Minus : Sum  Inputs=+-
  NOT : Logic  Operator=NOT  IconShape=distinctive  AllPortsSameDT=off  OutDataTypeStr=boolean
  NOT1 : Logic  Operator=NOT  IconShape=distinctive  AllPortsSameDT=off  OutDataTypeStr=boolean
  NOT2 : Logic  Operator=NOT  IconShape=distinctive  AllPortsSameDT=off  OutDataTypeStr=boolean
  OR : Logic  Operator=OR  IconShape=distinctive  AllPortsSameDT=off  OutDataTypeStr=boolean
  PID Controller : simulink/Continuous/PID Controller  Controller=PID  Form=Parallel  TimeDomain=Discrete-time  SampleTime=dt  IntegratorMethod=Forward Euler  FilterMethod=Forward Euler  ControllerParametersSource=internal  P=PowerError2Throttle  I=PowerErrorInt2Throttle  D=0  UseFilter=on  N=100  TunerSelectOption=Transfer Function Based (PID Tuner App)  InitialConditionSource=internal  InitialConditionForIntegrator=0  InitialConditionForFilter=0  DifferentiatorICPrevScaledInput=0  ExternalReset=level  TrackingMode=off  Kt=1  LimitOutput=off  UpperSaturationLimit=inf  LowerSaturationLimit=-inf  LinearizeAsGain=on  AntiWindupMode=none  Kb=1  POutMin=[]  POutMax=[]  IOutMin=[]  IOutMax=[]  DOutMin=[]  DOutMax=[]  NOutMin=[]  NOutMax=[]  SumOutMin=[]  SumOutMax=[]  SaturationOutMin=[]  SaturationOutMax=[]  PParamMin=[]  PParamMax=[]  IParamMin=[]  IParamMax=[]  DParamMin=[]  DParamMax=[]  NParamMin=[]  NParamMax=[]  KbParamMin=[]  KbParamMax=[]  KtParamMin=[]  KtParamMax=[]  KbOutMin=[]  KbOutMax=[]  KtOutMin=[]  KtOutMax=[]  IntegratorOutMin=[]  IntegratorOutMax=[]  FilterOutMin=[]  FilterOutMax=[]  SumI1OutMin=[]  SumI1OutMax=[]  SumI2OutMin=[]  SumI2OutMax=[]  SumI3OutMin=[]  SumI3OutMax=[]  SumI4OutMin=[]  SumI4OutMax=[]  SumDOutMin=[]  SumDOutMax=[]  DifferentiatorOutMin=[]  DifferentiatorOutMax=[]  FilterDiffOutCoefMin=[]  FilterDiffOutCoefMax=[]  ReciprocalOutMin=[]  ReciprocalOutMax=[]  SumDenOutMin=[]  SumDenOutMax=[]  SumNumOutMin=[]  SumNumOutMax=[]  DivideOutMin=[]  DivideOutMax=[]  IntegratorContinuousStateAttributes=''  IntegratorStateMustResolveToSignalObject=off  IntegratorRTWStateStorageClass=Auto  FilterContinuousStateAttributes=''  FilterStateMustResolveToSignalObject=off  FilterRTWStateStorageClass=Auto  ParallelPVariant=InternalParameters  IdealPVariant=Disabled  IVariant=InternalParameters  DVariant=InternalParameters  IntegratorVariant=Discrete  SatVariant=Disabled  AWVariant=Passthrough  PCopyVariant=Disabled  TRVariant=Disabled  FdbkBlocksVariant=Forward  IdealPFdbkVariant=Disabled  SatFdbkVariant=Disabled  DerivativeFilterVariant=ForwardEulerFilter  NVariant=InternalParameters  NCopyVariant=Disabled  FilterICVariant=InternalICsFilter  IntegratorICVariant=InternalICs  ExternalResetVariant=ExternalReset  TRSumVariant=Passthrough  SumFdbkVariant=Disabled  SumVariant=Sum_PID
  Rate Limiter Dynamic : simulink/Discontinuities/Rate Limiter Dynamic
      settings: SourceProductName=Simulink
  "Saturation " : Saturate  UpperLimit=ThrottleMax  LowerLimit=ThrottleMin  LinearizeAsGain=off
  Square : Math  Operator=square  SaturateOnIntegerOverflow=on
  Square1 : Math  Operator=square  SaturateOnIntegerOverflow=on
  Subsystem : Subsystem
  Sum : Sum  Inputs=|+-
  Sum1 : Sum  Inputs=++|
  Sum4 : Sum  Inputs=|++
  Sum5 : Sum  Inputs=|++
  Sum6 : Sum  Inputs=|++
  Switch{,1..3} (4 alike) : Switch  Criteria=u2 > Threshold  Threshold=0.5
  Throttle (Airspeed TEC) : Outport
  tag scope: AltErr=global, ThrottleCmd=global
  wires:
  Rate Limiter Dynamic/1 -> "Saturation "/1
  Vcmd/1 -> Square/1
  Square/1 -> Gain/1
  Divide/1 -> Gain1/1
  Gain1/1 -> Sum6/2
  Sum/1 -> "1/ MaxEnginePower "/1
  "1/ MaxEnginePower "/1 -> PID Controller/1  "Power Error"
  hCmd/1 -> Gain2/1, Minus/1
  Gain2/1 -> Sum4/1
  1st Order Reference Model/1(Rf) -> Sum/1
  Gain/1 -> 1st Order Reference Model/2(Vcmd), Sum4/2
  Square1/1 -> Gain3/1
  Gain3/1 -> Sum5/1
  Subsystem/1(Throttle Out) -> Switch1/3
  Bus Selector1/3 -> Divide/2  "<Vdot_mps2>"
  " "/1 -> Sum1/1
  "Saturation "/1 -> Throttle (Airspeed TEC)/1, [ThrottleCmd]  "Sim.Throttle (Airspeed)"
  Bus Selector1/1 -> Square1/1, Divide/1, 1st Order Reference Model/4("V ")  "<V_mps>"
  Bus Selector1/2 -> Gain7/1  "<hdot_m>"
  Feedback Bus/1 -> Bus Selector1/1
  Sum4/1 -> 1st Order Reference Model/1(Pcmd)
  Gain6/1 -> Sum5/2
  Sum5/1 -> 1st Order Reference Model/3(Pact)
  Gain7/1 -> Sum6/1
  Sum6/1 -> Sum/2
  Bus Selector1/4 -> Minus/2, Gain6/1  "<altitude_m>"
  Minus/1 -> [AltErr]
  " TLASaturation 1"/1 -> Subsystem/1(Throttle In)
  NOT1/1 -> Subsystem/2(Reset LPF)
  Switch2/1 -> Gain4/1, Rate Limiter Dynamic/1
  [pilotThr] -> Switch/3
  Constant3/1 -> Switch2/1
  Gain4/1 -> Rate Limiter Dynamic/3
  Switch/1 -> " TLASaturation 1"/1
  Constant5/1 -> Switch2/3
  [ApGlobal] -> Switch2/2, Switch/2, NOT1/1, NOT/1
  PID Controller/1 -> Sum1/2
  Sum1/1 -> Switch/1
  NOT/1 -> OR/1
  OR/1 -> PID Controller/2
  NOT2/1 -> OR/2
  [Flag_TAS_Priority] -> NOT2/1
  [Flag_Underspeed] -> AND/1
  [ApGlobal] -> AND/2
  AND/1 -> Switch1/2
  Switch1/1 -> Switch3/3
  Constant/1 -> Switch1/1
  Switch3/1 -> Rate Limiter Dynamic/2
  AND1/1 -> Switch3/2
  [Flag_Overspeed] -> AND1/1
  [ApGlobal] -> AND1/2
  Constant1/1 -> Switch3/1
